simulink model "carboncycle"  (R2020a)
settings: Solver=VariableStepAuto  StartTime=0.0  StopTime=10  RelTol=1e-6
model workspace (MAT data in the model file):
  c_forest_burning_biofuel_co2_released = 1.85
  c_forest_burning_biofuel_energy_released = 4519.72
  c_forest_burning_co2_released = [0.9792 0.9792 2.52 2.52 2.52 2.52 2.52 3.6]
  c_forest_burning_energy_released = [1167.1928 1167.1928 1485.04 1485.04 1485.04 1485.04 1398.78 1398.78]
  c_forest_burning_losses_co2_released = [1.76436 1.76436 0 0 0 0 0 0]
  c_forest_burning_losses_energy_released = [1974.86 1974.86 0 0 0 0 0 0]
  c_harvesting = 1.13940256046
  c_production_biofuel_cost_co2 = 0.74
  c_production_biofuel_cost_tall_oil = 1
  c_production_co2_forest = [0.031 1.667745 0.37375 0.37375 0.37375 0.37375 0.37375 1.1]
  c_production_co2_substitute = [1.539 1.539 1.384806222 1.738255325 12.95940153 13.79703167 0 0]
  c_production_losses_used_for_biofuel = [0 0 0.005521208 0.005521208 0.005521208 0.005521208 0.005521208 0.005521208]
  c_production_losses_used_for_energy = [0.136 0.136 0 0 0 0 0 0]
  c_production_pulp_raw_wood_demand = 3.2229
  c_production_pulp_used = [0 0 1 1 1 1 1 1]
  c_production_pulp_used_reciprocal = [0 0 1 1 1 1 1 1]
  c_production_raw_wood = [2 2 3.2229 3.2229 3.2229 3.2229 3.2229 3.2229]
  c_production_raw_wood_used = [1 1 0 0 0 0 0 0]
  c_production_to_pulp = [0.8 0.8 0 0 0 0 0 0]
  c_recycling_co2_forest = [0 0 1.05 1.05 1.05 1.05 1.05 0]
  c_recycling_co2_substitute = [2.214338235 2.214338235 1.864705882 2.097794118 8.55 0.156 0 0]
  c_substitute_burning_co2_released = [2.922732 2.922732 2.465568 2.773764 0 0 0 0]
  c_substitute_burning_energy_released = [4004.212 4004.212 3616.688 3793.464 0 0 0 0]
  convert_co2_to_forestvolume = 1
  forest_age_0 = 61.5
  forest_area = 20276000
  forest_volume_0 = 2409000000
  initial_stock = 86700000
  k_autotrophic_respiration = 0.5
  k_energy_recovery_forest = [1; 1; 0.070939484; 0.070939484; 0.070939484; 0.070939484; 0.070939484; 1]
  k_energy_recovery_substitute = [0.360473602; 0.360473602; 0.360473602; 0.360473602; 0.111618603; 0; 0; 0]
  k_final_felling = 0.0342
  k_heterotrophic_respiration = 0.5
  k_incineration_forest = [0; 0; 0; 0; 0; 0; 0; 0]
  k_incineration_substitute = [0.008399732; 0.008399732; 0.008399732; 0.008399732; 0.001222426; 0.001; 1; 1]
  k_material_recovery_forest = [0; 0; 0.929060516; 0.929060516; 0.929060516; 0.929060516; 0.929060516; 0]
  k_material_recovery_substitute = [0.631126662; 0.631126662; 0.631126662; 0.631126662; 0.887158971; 0.999; 0; 0]
  k_natural_loss = 0.00227171311509
  k_sustainable_harvesting = 0.03
  k_waste_co2_release_forest = 1
  k_waste_co2_release_substitute = 1
  max_forest = 7227000000
libraries: simulink x3
settings Model: OrderedModelArguments=off  Creator=Cosmo  LastModifiedBy=Roni
settings SolverCC: AlgebraicLoopSolver=LineSearch
settings DataIOCC: SaveFormat=StructureWithTime  SignalLogging=off  DSMLogging=off  SaveTime=off
settings DebuggingCC: ArithmeticOperatorsInVariantConditions=warning
settings SFSimCC: CustomCodeUndefinedFunction=UseInterfaceOnly

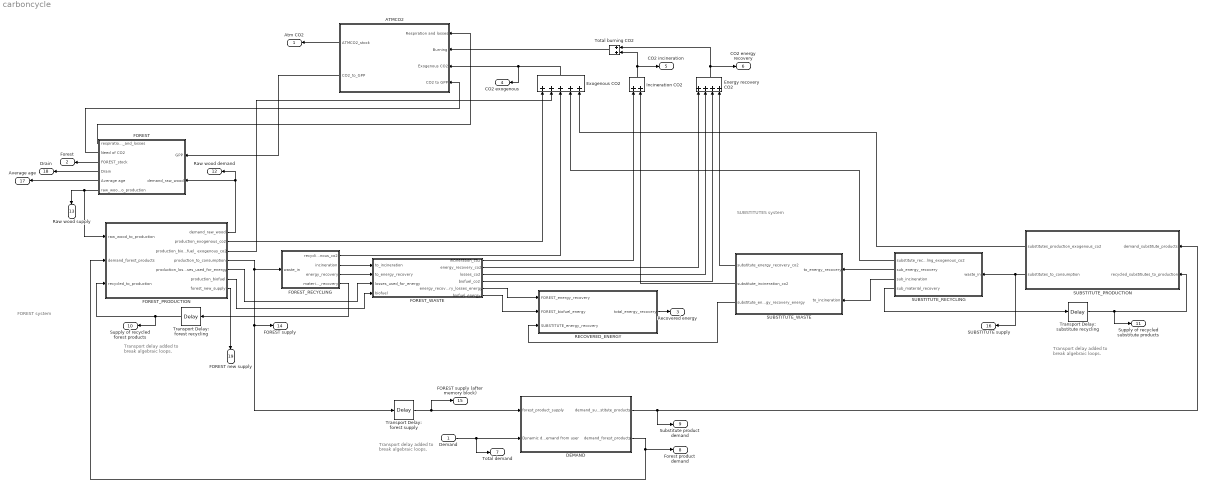
== system carboncycle ==
  note: Transport delay added
      | to break algebraic loops.
  note: FOREST system
  note: SUBSTITUTES system
  note: Transport delay
      | added
      | to break algebraic loops.
  note: Transport delay added
      | to break algebraic loops.
  Demand : Inport  PortDimensions=8
  ATMCO2 : Subsystem
  DEMAND : Subsystem
  Energy recovery CO2 : Sum  Inputs=++++
  Exogenous CO2 : Sum  Inputs=+++++
  FOREST : Subsystem
  FOREST_PRODUCTION : Subsystem
  FOREST_RECYCLING : Subsystem
  FOREST_WASTE : Subsystem
  Incineration CO2 : Sum
  RECOVERED_ENERGY : Subsystem
  SUBSTITUTE_PRODUCTION : Subsystem
  SUBSTITUTE_RECYCLING : Subsystem
  SUBSTITUTE_WASTE : Subsystem
  Total burning CO2 : Sum
  Transport Delay: forest recycling : TransportDelay  DelayTime=0.1
  Transport Delay: forest supply : TransportDelay  DelayTime=0.1
  Transport Delay: substitute recycling : TransportDelay  DelayTime=0.1
  Atm CO2 : Outport
  Forest : Outport  Port=2  Unit=m^3
  Recovered energy : Outport  Port=3
  CO2 exogenous : Outport  Port=4
  CO2 incineration : Outport  Port=5
  CO2 energy recovery : Outport  Port=6
  Total demand : Outport  Port=7
  Forest product demand : Outport  Port=8
  Substitute product demand : Outport  Port=9
  Supply of recycled forest products : Outport  Port=10
  Supply of recycled substitute products : Outport  Port=11
  Raw wood demand : Outport  Port=12
  Raw wood supply : Outport  Port=13
  FOREST supply : Outport  Port=14
  FOREST supply (after memory block) : Outport  Port=15
  SUBSTITUTE supply : Outport  Port=16
  Average age : Outport  Port=17
  Drain : Outport  Port=18  Unit=m^3
  FOREST new supply : Outport  Port=19
  wires:
  ATMCO2/2(CO2_to_GPP) -> FOREST/1(GPP)
  FOREST/1(respiration_and_losses) -> ATMCO2/1(Respiration and losses)
  FOREST/6(raw_wood_to_production) -> Raw wood supply/1, FOREST_PRODUCTION/1(raw_wood_to_production)
  FOREST_RECYCLING/4(material_recovery) -> Transport Delay: forest recycling/1
  FOREST_RECYCLING/1(recycling_exogenous_co2) -> Exogenous CO2/3
  FOREST_PRODUCTION/2(production_exogenous_co2) -> Exogenous CO2/1
  DEMAND/2(demand_forest_products) -> Forest product demand/1, FOREST_PRODUCTION/2(demand_forest_products)
  SUBSTITUTE_PRODUCTION/2(substitutes_to_consumption) -> SUBSTITUTE_RECYCLING/1(waste_in), SUBSTITUTE supply/1
  SUBSTITUTE_RECYCLING/1(substitute_recycling_exogenous_co2) -> Exogenous CO2/4
  SUBSTITUTE_PRODUCTION/1(substitutes_production_exogenous_co2) -> Exogenous CO2/5
  SUBSTITUTE_WASTE/1(substitute_energy_recovery_co2) -> Energy recovery CO2/4
  SUBSTITUTE_RECYCLING/4(sub_material_recovery) -> Transport Delay: substitute recycling/1
  FOREST/2(Need of CO2) -> ATMCO2/4(CO2 to GPP)
  FOREST_RECYCLING/2(incineration) -> FOREST_WASTE/1(to_incineration)
  FOREST_RECYCLING/3(energy_recovery) -> FOREST_WASTE/2(to_energy_recovery)
  FOREST_WASTE/1(incineration_co2) -> Incineration CO2/1
  FOREST_WASTE/5(energy_recovery_losses_energy) -> RECOVERED_ENERGY/1(FOREST_energy_recovery)
  RECOVERED_ENERGY/1(total_energy_recovery) -> Recovered energy/1
  SUBSTITUTE_WASTE/3(substitute_energy_recovery_energy) -> RECOVERED_ENERGY/3(SUBSTITUTE_energy_recovery)
  FOREST_WASTE/2(energy_recovery_co2) -> Energy recovery CO2/1
  Incineration CO2/1 -> CO2 incineration/1, Total burning CO2/2
  Total burning CO2/1 -> ATMCO2/2(Burning)
  SUBSTITUTE_RECYCLING/2(sub_energy_recovery) -> SUBSTITUTE_WASTE/1(to_energy_recovery)
  SUBSTITUTE_RECYCLING/3(sub_incineration) -> SUBSTITUTE_WASTE/2(to_incineration)
  Transport Delay: forest recycling/1 -> Supply of recycled forest products/1, FOREST_PRODUCTION/3(recycled_to_production)
  Energy recovery CO2/1 -> CO2 energy recovery/1, Total burning CO2/1
  Exogenous CO2/1 -> CO2 exogenous/1, ATMCO2/3(Exogenous CO2)
  Transport Delay: forest supply/1 -> FOREST supply (after memory block)/1, DEMAND/1(forest_product_supply)
  FOREST_PRODUCTION/4(production_to_consumption) -> Transport Delay: forest supply/1, FOREST supply/1, FOREST_RECYCLING/1(waste_in)
  Transport Delay: substitute recycling/1 -> Supply of recycled substitute products/1, SUBSTITUTE_PRODUCTION/2(recycled_substitiutes_to_production)
  FOREST/3(FOREST_stock) -> Forest/1
  ATMCO2/1(ATMCO2_stock) -> Atm CO2/1
  FOREST_PRODUCTION/1(demand_raw_wood) -> Raw wood demand/1, FOREST/2(demand_raw_wood)
  FOREST_PRODUCTION/5(production_losses_used_for_energy) -> FOREST_WASTE/3(losses_used_for_energy)
  FOREST_PRODUCTION/6(production_biofuel) -> FOREST_WASTE/4(biofuel)
  FOREST_PRODUCTION/3(production_biofuel_ exogenous_co2) -> Exogenous CO2/2
  FOREST_WASTE/6(biofuel_energy) -> RECOVERED_ENERGY/2(FOREST_biofuel_energy)
  FOREST_WASTE/3(losses_co2) -> Energy recovery CO2/2
  FOREST_WASTE/4(biofuel_co2) -> Energy recovery CO2/3
  SUBSTITUTE_WASTE/2(substitute_incineration_co2) -> Incineration CO2/2
  FOREST/5(Average age) -> Average age/1
  FOREST/4(Drain) -> Drain/1
  DEMAND/1(demand_substitute_products) -> Substitute product demand/1, SUBSTITUTE_PRODUCTION/1(demand_substitute_products)
  Demand/1 -> Total demand/1, DEMAND/2(Dynamic demand from user)
  FOREST_PRODUCTION/7(forest_new_supply) -> FOREST new supply/1

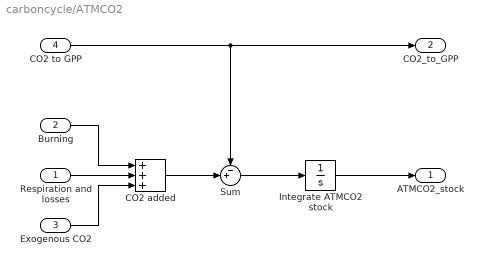
== system carboncycle/ATMCO2 ==
  Respiration and losses : Inport
  Burning : Inport  Port=2
  Exogenous CO2 : Inport  Port=3  Unit=t
  CO2 to GPP : Inport  Port=4  Unit=t
  CO2 added : Sum  Inputs=+++
  Integrate ATMCO2 stock : Integrator
  Sum : Sum  Inputs=-+|
  ATMCO2_stock : Outport  Unit=t
  CO2_to_GPP : Outport  Port=2  Unit=t
  wires:
  Burning/1 -> CO2 added/1
  Respiration and losses/1 -> CO2 added/2
  Exogenous CO2/1 -> CO2 added/3
  Integrate ATMCO2 stock/1 -> ATMCO2_stock/1
  Sum/1 -> Integrate ATMCO2 stock/1
  CO2 added/1 -> Sum/2
  CO2 to GPP/1 -> Sum/1, CO2_to_GPP/1

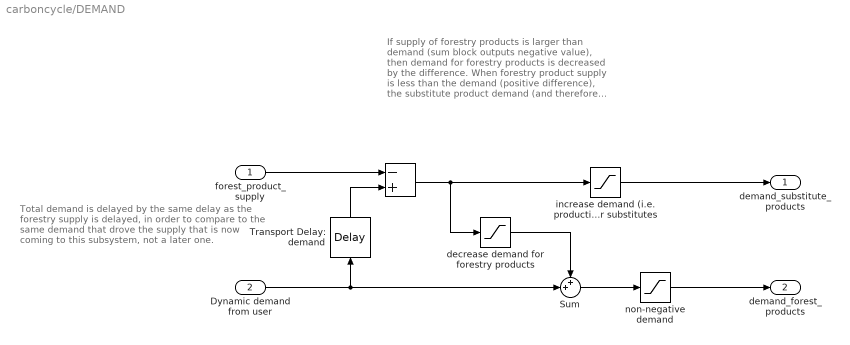
== system carboncycle/DEMAND ==
  note: If supply of forestry products is larger than demand (sum block outputs negative value), then demand for forestry products is decreased by the difference.
      |
      | When forestry product supply is less than the demand (positive difference), the substitute product demand (and therefore production) is equal to this difference.
  note: Total demand is delayed by the same delay as the forestry supply is delayed, in order to compare to the same demand that drove the supply that is now coming to this subsystem, not a later one.
  forest_product_supply : Inport
  Dynamic demand from user : Inport  Port=2
  " " : Sum  Inputs=-+
  Sum : Sum  Inputs=++|
  Transport Delay: demand : TransportDelay  DelayTime=0.1
  decrease demand for forestry products : Saturate  UpperLimit=0  LowerLimit=-inf  ZeroCross=off
  increase demand (i.e. production) for substitutes : Saturate  UpperLimit=inf  LowerLimit=0  ZeroCross=off
  non-negative demand : Saturate  UpperLimit=inf  LowerLimit=0
  demand_substitute_products : Outport
  demand_forest_products : Outport  Port=2
  wires:
  " "/1 -> decrease demand for forestry products/1, increase demand (i.e. production) for substitutes/1
  decrease demand for forestry products/1 -> Sum/1
  Sum/1 -> non-negative demand/1
  forest_product_supply/1 -> " "/1
  Dynamic demand from user/1 -> Sum/2, Transport Delay: demand/1
  non-negative demand/1 -> demand_forest_products/1
  increase demand (i.e. production) for substitutes/1 -> demand_substitute_products/1
  Transport Delay: demand/1 -> " "/2

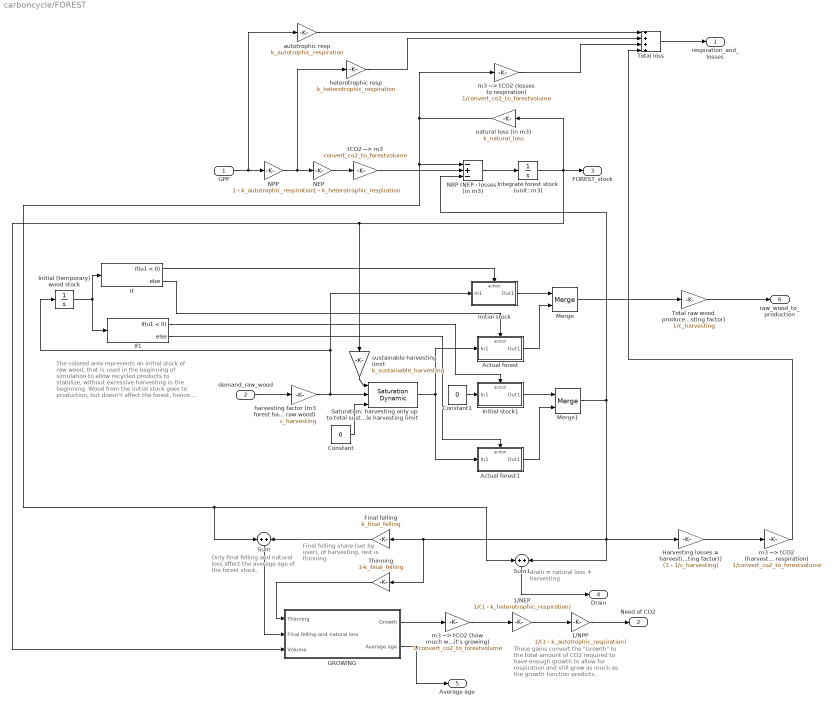
== system carboncycle/FOREST ==
  note: drain =
      | natural loss
      | + harvesting
  note: Final felling share (set
      | by user), of harvesting,
      | rest is thinning.
  note: The colored area represents an initial stock of raw wood, that is used in the beginning of simulation to allow recycled products to stabilize, without excessive harvesting in the beginning. Wood from the initial stock goes to production, but doesn't affect the forest, hence different merge blocks.
      |
      | After the initial stock is empty (i.e. u1 > 0), we start to harvest the actual forest.
  note: Only final felling
      | and natural loss
      | affect the average
      | age of the forest
      | stock.
  note: These gains convert the "Growth"
      | to the total amount of CO2 required
      | to have enough growth to allow for
      | respiration and still grow as much as
      | the growth function predicts.
  GPP : Inport
  demand_raw_wood : Inport  Port=2  Unit=m^3
  1/NEP : Gain  Gain=1/(1 - k_heterotrophic_respiration)
  1/NPP : Gain  Gain=1/(1 - k_autotrophic_respiration)
  Actual forest : Subsystem  TreatAsAtomicUnit=on
  Actual forest1 : Subsystem  TreatAsAtomicUnit=on
  Constant : Constant  Value=0
  Constant1 : Constant  Value=0
  Final felling : Gain  Gain=k_final_felling
  GROWING : Subsystem
  Harvesting losses = harvesting * (1 - 1 / (harvesting factor)) : Gain  Gain=(1 - 1/c_harvesting)
  If : If  IfExpression=u1 < 0  ZeroCross=off
  If1 : If  IfExpression=u1 < 0  ZeroCross=off
  Initial (temporary) wood stock : Integrator  InitialCondition=-initial_stock
  Initial stock : Subsystem  TreatAsAtomicUnit=on
  Initial stock1 : Subsystem  TreatAsAtomicUnit=on
  Integrate forest stock (unit: m3) : Integrator  InitialCondition=forest_volume_0
  Merge : Merge
  Merge1 : Merge
  NBP (NEP - losses) (in m3) : Sum  Inputs=-+-
  NEP : Gain  Gain=1 - k_heterotrophic_respiration
  NPP : Gain  Gain=1 - k_autotrophic_respiration
  Saturation: harvesting only up to total sustainable harvesting limit : simulink/Discontinuities/Saturation Dynamic  OutMin=[]  OutMax=[]  OutDataTypeStr=Inherit: Same as second input  OutDataType=fixdt(1, 16)  OutScaling=2^-10  DoSatur=off
  Sum : Sum  Inputs=+|+
  Sum1 : Sum  Inputs=+|+
  Thinning : Gain  Gain=1-k_final_felling
  Total loss : Sum  Inputs=++++
  Total raw wood produced = harvesting / (harvesting factor) : Gain  Gain=1/c_harvesting
  autotrophic resp : Gain  Gain=k_autotrophic_respiration
  harvesting factor (m3 forest harvested for m3 raw wood) : Gain  Gain=c_harvesting
  heterotrophic resp : Gain  Gain=k_heterotrophic_respiration
  m3 --> tCO2 (harvesting losses to respiration) : Gain  Gain=1/convert_co2_to_forestvolume
  m3 --> tCO2 (how much wood absorbs CO2 when it's growing) : Gain  Gain=1/convert_co2_to_forestvolume
  m3 --> tCO2 (losses to respiration) : Gain  Gain=1/convert_co2_to_forestvolume
  natural loss (in m3) : Gain  Gain=k_natural_loss
  sustainable harvesting limit : Gain  Gain=k_sustainable_harvesting
  tCO2 --> m3 : Gain  Gain=convert_co2_to_forestvolume
  respiration_and_losses : Outport  Unit=t
  Need of CO2 : Outport  Port=2  Unit=t  VectorParamsAs1DForOutWhenUnconnected=off
  FOREST_stock : Outport  Port=3  Unit=m^3
  Drain : Outport  Port=4  Unit=m^3
  Average age : Outport  Port=5  Unit=y  VectorParamsAs1DForOutWhenUnconnected=off
  raw_wood_to_production : Outport  Port=6  Unit=m^3
  wires:
  GPP/1 -> autotrophic resp/1, NPP/1
  NPP/1 -> heterotrophic resp/1, NEP/1
  NEP/1 -> tCO2 --> m3/1
  autotrophic resp/1 -> Total loss/1
  heterotrophic resp/1 -> Total loss/2
  Total loss/1 -> respiration_and_losses/1
  NBP (NEP - losses) (in m3)/1 -> Integrate forest stock (unit: m3)/1
  natural loss (in m3)/1 -> Sum1/1, Sum/1, NBP (NEP - losses) (in m3)/1, m3 --> tCO2 (losses to respiration)/1
  demand_raw_wood/1 -> harvesting factor (m3 forest harvested for m3 raw wood)/1
  Total raw wood produced = harvesting / (harvesting factor)/1 -> raw_wood_to_production/1
  tCO2 --> m3/1 -> NBP (NEP - losses) (in m3)/2
  m3 --> tCO2 (losses to respiration)/1 -> Total loss/3
  Harvesting losses = harvesting * (1 - 1 / (harvesting factor))/1 -> m3 --> tCO2 (harvesting losses to respiration)/1
  m3 --> tCO2 (harvesting losses to respiration)/1 -> Total loss/4
  m3 --> tCO2 (how much wood absorbs CO2 when it's growing)/1 -> 1/NEP/1
  1/NPP/1 -> Need of CO2/1
  1/NEP/1 -> 1/NPP/1
  GROWING/1("Growth ") -> m3 --> tCO2 (how much wood absorbs CO2 when it's growing)/1
  Integrate forest stock (unit: m3)/1 -> natural loss (in m3)/1, FOREST_stock/1, sustainable harvesting limit/1, GROWING/3(Volume)
  Thinning/1 -> GROWING/1(Thinning)
  Sum/1 -> GROWING/2("Final felling and natural loss ")
  Final felling/1 -> Sum/2
  GROWING/2(Average age) -> Average age/1
  Constant/1 -> Saturation: harvesting only up to total sustainable harvesting limit/3
  harvesting factor (m3 forest harvested for m3 raw wood)/1 -> Initial (temporary) wood stock/1, Initial stock/1(In1), Saturation: harvesting only up to total sustainable harvesting limit/2
  Initial (temporary) wood stock/1 -> If/1, If1/1
  sustainable harvesting limit/1 -> Saturation: harvesting only up to total sustainable harvesting limit/1
  If/1 -> Initial stock/Action
  If/2 -> Actual forest/Action
  Saturation: harvesting only up to total sustainable harvesting limit/1 -> Actual forest/1(In1), Actual forest1/1(In1)
  Initial stock/1(Out1) -> Merge/1
  Merge/1 -> Total raw wood produced = harvesting / (harvesting factor)/1
  Actual forest/1(Out1) -> Merge/2
  Merge1/1 -> NBP (NEP - losses) (in m3)/3, Thinning/1, Final felling/1, Sum1/2, Harvesting losses = harvesting * (1 - 1 / (harvesting factor))/1
  Actual forest1/1(Out1) -> Merge1/2
  Initial stock1/1(Out1) -> Merge1/1
  If1/1 -> Initial stock1/Action
  Constant1/1 -> Initial stock1/1(In1)
  If1/2 -> Actual forest1/Action
  Sum1/1 -> Drain/1

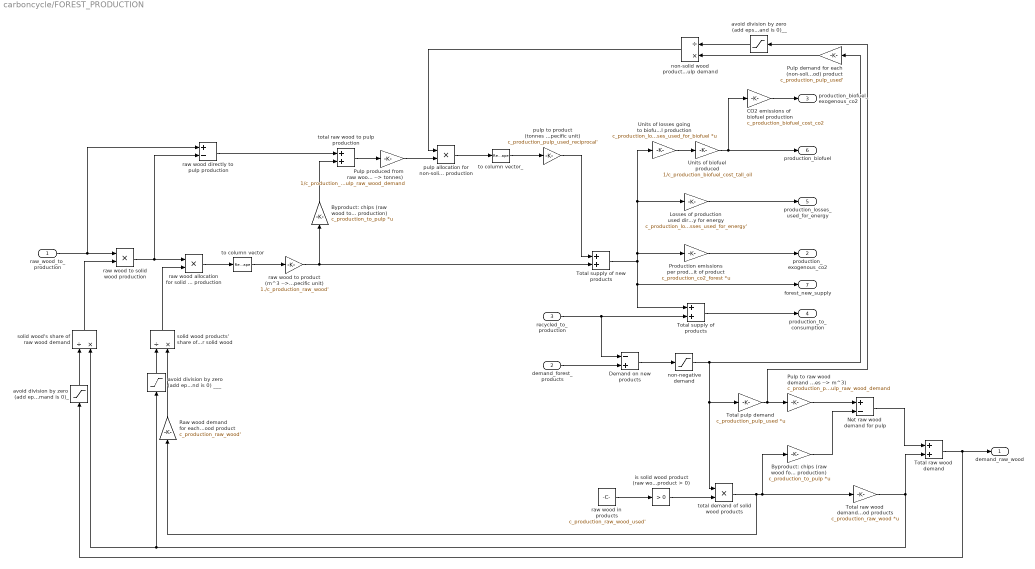
== system carboncycle/FOREST_PRODUCTION ==
  raw_wood_to_production : Inport  Unit=m^3
  demand_forest_products : Inport  Port=2
  recycled_to_production : Inport  Port=3
  Byproduct: chips (raw wood for pulp production) : Gain  Gain=c_production_to_pulp  Multiplication=Matrix(K*u)
  Byproduct: chips (raw wood to pulp production) : Gain  Gain=c_production_to_pulp  Multiplication=Matrix(K*u)
  CO2 emissions of biofuel production : Gain  Gain=c_production_biofuel_cost_co2
  Demand on new products : Sum  Inputs=-+
  Losses of production used directly for energy : Gain  Gain=c_production_losses_used_for_energy'
  Net raw wood demand for pulp : Sum  Inputs=+-
  Production emissions per produced unit of product : Gain  Gain=c_production_co2_forest  Multiplication=Matrix(K*u)
  Pulp demand for each (non-solid wood) product : Gain  Gain=c_production_pulp_used'
  Pulp produced from raw wood (m^3 --> tonnes) : Gain  Gain=1/c_production_pulp_raw_wood_demand
  Pulp to raw wood demand (tonnes --> m^3) : Gain  Gain=c_production_pulp_raw_wood_demand
  Raw wood demand for each solid wood product : Gain  Gain=c_production_raw_wood'
  Total pulp demand : Gain  Gain=c_production_pulp_used  Multiplication=Matrix(K*u)
  Total raw wood demand : Sum
  Total raw wood demand for solid wood products : Gain  Gain=c_production_raw_wood  Multiplication=Matrix(K*u)
  Total supply of new products : Sum
  Total supply of products : Sum
  Units of biofuel produced : Gain  Gain=1/c_production_biofuel_cost_tall_oil
  Units of losses going to biofuel production : Gain  Gain=c_production_losses_used_for_biofuel  Multiplication=Matrix(K*u)
  avoid division by zero (add eps if total demand is 0)_ : Saturate  UpperLimit=Inf  LowerLimit=eps
  avoid division by zero (add eps if total demand is 0)__ : Saturate  UpperLimit=Inf  LowerLimit=eps
  avoid division by zero (add eps if total demand is 0) ___ : Saturate  UpperLimit=Inf  LowerLimit=eps
  is solid wood product (raw wood in product > 0) : simulink/Logic and Bit Operations/Compare To Zero  relop=>  OutDataTypeStr=boolean
  non-negative demand : Saturate  UpperLimit=Inf  LowerLimit=0
  non-solid wood products' share of pulp demand : Product  Inputs=/*  OutMin=0  OutMax=1
  pulp allocation for non-solid wood production : Product
  pulp to product (tonnes --> product- specific unit) : Gain  Gain=c_production_pulp_used_reciprocal'
  raw wood allocation for solid wood production : Product
  raw wood directly to pulp production : Sum  Inputs=+-
  raw wood in products : Constant  Value=c_production_raw_wood_used'
  raw wood to product (m^3 --> product-specific unit) : Gain  Gain=1./c_production_raw_wood'
  raw wood to solid wood production : Product
  solid wood products' share of raw wood demand for solid wood : Product  Inputs=/*  OutMin=0  OutMax=1
  solid wood's share of raw wood demand : Product  Inputs=/*  OutMin=0  OutMax=1
  to column vector : Reshape  OutputDimensionality=Column vector (2-D)
  to column vector_ : Reshape  OutputDimensionality=Column vector (2-D)
  total demand of solid wood products : Product  OutDataTypeStr=double
  total raw wood to pulp production : Sum
  demand_raw_wood : Outport  Unit=m^3
  production_exogenous_co2 : Outport  Port=2  Unit=t
  production_biofuel_ exogenous_co2 : Outport  Port=3  Unit=t
  production_to_consumption : Outport  Port=4
  production_losses_used_for_energy : Outport  Port=5
  production_biofuel : Outport  Port=6
  forest_new_supply : Outport  Port=7
  wires:
  Production emissions per produced unit of product/1 -> production_exogenous_co2/1
  Total supply of products/1 -> production_to_consumption/1
  raw_wood_to_production/1 -> raw wood to solid wood production/1, raw wood directly to pulp production/1
  Demand on new products/1 -> non-negative demand/1
  demand_forest_products/1 -> Demand on new products/2
  recycled_to_production/1 -> Demand on new products/1, Total supply of products/2
  non-negative demand/1 -> total demand of solid wood products/1, Total pulp demand/1, Pulp demand for each (non-solid wood) product/1
  is solid wood product (raw wood in product > 0)/1 -> total demand of solid wood products/2
  raw wood in products/1 -> is solid wood product (raw wood in product > 0)/1
  total demand of solid wood products/1 -> Byproduct: chips (raw wood for pulp production)/1, Total raw wood demand for solid wood products/1, Raw wood demand for each solid wood product/1
  Total pulp demand/1 -> avoid division by zero (add eps if total demand is 0)__/1, Pulp to raw wood demand (tonnes --> m^3)/1
  Pulp to raw wood demand (tonnes --> m^3)/1 -> Net raw wood demand for pulp/1
  Byproduct: chips (raw wood for pulp production)/1 -> Net raw wood demand for pulp/2
  Net raw wood demand for pulp/1 -> Total raw wood demand/1
  Total raw wood demand for solid wood products/1 -> Total raw wood demand/2, solid wood's share of raw wood demand/2, avoid division by zero (add eps if total demand is 0) ___/1
  Total raw wood demand/1 -> avoid division by zero (add eps if total demand is 0)_/1, demand_raw_wood/1
  avoid division by zero (add eps if total demand is 0)_/1 -> solid wood's share of raw wood demand/1
  solid wood's share of raw wood demand/1 -> raw wood to solid wood production/2
  raw wood to solid wood production/1 -> raw wood allocation for solid wood production/1, raw wood directly to pulp production/2
  raw wood to product (m^3 --> product-specific unit)/1 -> Total supply of new products/2, Byproduct: chips (raw wood to pulp production)/1
  Byproduct: chips (raw wood to pulp production)/1 -> total raw wood to pulp production/2
  raw wood directly to pulp production/1 -> total raw wood to pulp production/1
  Raw wood demand for each solid wood product/1 -> solid wood products' share of raw wood demand for solid wood/2
  avoid division by zero (add eps if total demand is 0) ___/1 -> solid wood products' share of raw wood demand for solid wood/1
  solid wood products' share of raw wood demand for solid wood/1 -> raw wood allocation for solid wood production/2
  raw wood allocation for solid wood production/1 -> to column vector/1
  total raw wood to pulp production/1 -> Pulp produced from raw wood (m^3 --> tonnes)/1
  pulp to product (tonnes --> product- specific unit)/1 -> Total supply of new products/1
  to column vector/1 -> raw wood to product (m^3 --> product-specific unit)/1
  Pulp produced from raw wood (m^3 --> tonnes)/1 -> pulp allocation for non-solid wood production/2
  pulp allocation for non-solid wood production/1 -> to column vector_/1
  to column vector_/1 -> pulp to product (tonnes --> product- specific unit)/1
  avoid division by zero (add eps if total demand is 0)__/1 -> non-solid wood products' share of pulp demand/1
  Pulp demand for each (non-solid wood) product/1 -> non-solid wood products' share of pulp demand/2
  non-solid wood products' share of pulp demand/1 -> pulp allocation for non-solid wood production/1
  Losses of production used directly for energy/1 -> production_losses_used_for_energy/1
  Units of losses going to biofuel production/1 -> Units of biofuel produced/1
  Total supply of new products/1 -> Units of losses going to biofuel production/1, Losses of production used directly for energy/1, Production emissions per produced unit of product/1, Total supply of products/1, forest_new_supply/1
  Units of biofuel produced/1 -> CO2 emissions of biofuel production/1, production_biofuel/1
  CO2 emissions of biofuel production/1 -> production_biofuel_ exogenous_co2/1

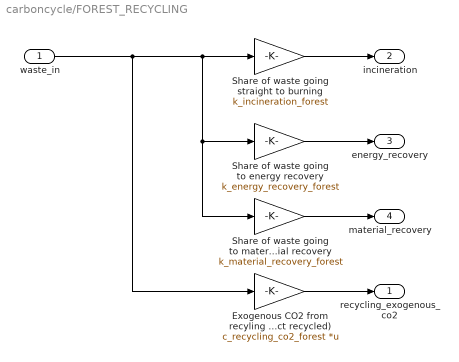
== system carboncycle/FOREST_RECYCLING ==
  waste_in : Inport
  Exogenous CO2 from recyling (tCO2 / unit of product recycled) : Gain  Gain=c_recycling_co2_forest  Multiplication=Matrix(K*u)
  Share of waste going straight to burning : Gain  Gain=k_incineration_forest
  Share of waste going to energy recovery : Gain  Gain=k_energy_recovery_forest
  Share of waste going to material recovery : Gain  Gain=k_material_recovery_forest
  recycling_exogenous_co2 : Outport  Unit=t
  incineration : Outport  Port=2
  energy_recovery : Outport  Port=3
  material_recovery : Outport  Port=4
  wires:
  Share of waste going to material recovery/1 -> material_recovery/1
  Exogenous CO2 from recyling (tCO2 / unit of product recycled)/1 -> recycling_exogenous_co2/1
  Share of waste going to energy recovery/1 -> energy_recovery/1
  waste_in/1 -> Exogenous CO2 from recyling (tCO2 / unit of product recycled)/1, Share of waste going to energy recovery/1, Share of waste going to material recovery/1, Share of waste going straight to burning/1
  Share of waste going straight to burning/1 -> incineration/1

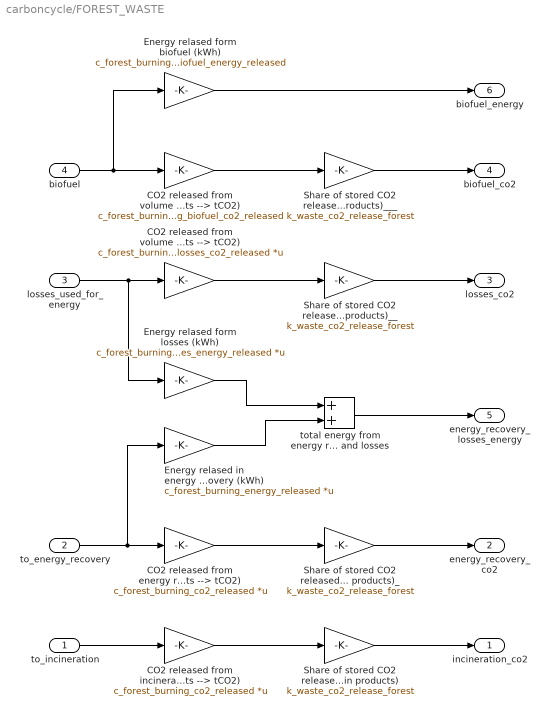
== system carboncycle/FOREST_WASTE ==
  to_incineration : Inport
  to_energy_recovery : Inport  Port=2
  losses_used_for_energy : Inport  Port=3
  biofuel : Inport  Port=4
  CO2 released from energy recovery volume (product units --> tCO2) : Gain  Gain=c_forest_burning_co2_released  Multiplication=Matrix(K*u)
  CO2 released from incineration volume (product units --> tCO2) : Gain  Gain=c_forest_burning_co2_released  Multiplication=Matrix(K*u)
  CO2 released from volume of biofuel (biofuel units --> tCO2) : Gain  Gain=c_forest_burning_biofuel_co2_released
  CO2 released from volume of losses used for energy (loss units --> tCO2) : Gain  Gain=c_forest_burning_losses_co2_released  Multiplication=Matrix(K*u)
  Energy relased form biofuel (kWh) : Gain  Gain=c_forest_burning_biofuel_energy_released
  Energy relased form losses (kWh) : Gain  Gain=c_forest_burning_losses_energy_released  Multiplication=Matrix(K*u)
  Energy relased in energy recovery (kWh) : Gain  Gain=c_forest_burning_energy_released  Multiplication=Matrix(K*u)
  Share of stored CO2 released through burning (tCO2 / tCO2 stored in products) : Gain  Gain=k_waste_co2_release_forest
  Share of stored CO2 released through burning (tCO2 / tCO2 stored in products)_ : Gain  Gain=k_waste_co2_release_forest
  Share of stored CO2 released through burning (tCO2 / tCO2 stored in products)__ : Gain  Gain=k_waste_co2_release_forest
  Share of stored CO2 released through burning (tCO2 / tCO2 stored in products)___ : Gain  Gain=k_waste_co2_release_forest
  total energy from energy recovery and losses : Sum
  incineration_co2 : Outport  Unit=t
  energy_recovery_co2 : Outport  Port=2  Unit=t
  losses_co2 : Outport  Port=3  Unit=t
  biofuel_co2 : Outport  Port=4  Unit=t
  energy_recovery_losses_energy : Outport  Port=5  Unit=kWh
  biofuel_energy : Outport  Port=6  Unit=kWh
  wires:
  CO2 released from incineration volume (product units --> tCO2)/1 -> Share of stored CO2 released through burning (tCO2 / tCO2 stored in products)/1
  Share of stored CO2 released through burning (tCO2 / tCO2 stored in products)/1 -> incineration_co2/1
  to_energy_recovery/1 -> CO2 released from energy recovery volume (product units --> tCO2)/1, Energy relased in energy recovery (kWh)/1
  to_incineration/1 -> CO2 released from incineration volume (product units --> tCO2)/1
  CO2 released from energy recovery volume (product units --> tCO2)/1 -> Share of stored CO2 released through burning (tCO2 / tCO2 stored in products)_/1
  Share of stored CO2 released through burning (tCO2 / tCO2 stored in products)_/1 -> energy_recovery_co2/1
  losses_used_for_energy/1 -> Energy relased form losses (kWh)/1, CO2 released from volume of losses used for energy (loss units --> tCO2)/1
  CO2 released from volume of losses used for energy (loss units --> tCO2)/1 -> Share of stored CO2 released through burning (tCO2 / tCO2 stored in products)__/1
  CO2 released from volume of biofuel (biofuel units --> tCO2)/1 -> Share of stored CO2 released through burning (tCO2 / tCO2 stored in products)___/1
  biofuel/1 -> Energy relased form biofuel (kWh)/1, CO2 released from volume of biofuel (biofuel units --> tCO2)/1
  Share of stored CO2 released through burning (tCO2 / tCO2 stored in products)___/1 -> biofuel_co2/1
  Share of stored CO2 released through burning (tCO2 / tCO2 stored in products)__/1 -> losses_co2/1
  Energy relased in energy recovery (kWh)/1 -> total energy from energy recovery and losses/2
  Energy relased form losses (kWh)/1 -> total energy from energy recovery and losses/1
  total energy from energy recovery and losses/1 -> energy_recovery_losses_energy/1
  Energy relased form biofuel (kWh)/1 -> biofuel_energy/1

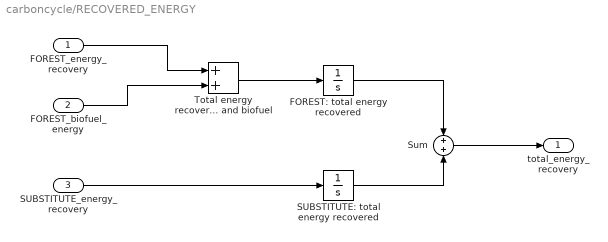
== system carboncycle/RECOVERED_ENERGY ==
  FOREST_energy_recovery : Inport  Unit=kWh
  FOREST_biofuel_energy : Inport  Port=2  Unit=kWh
  SUBSTITUTE_energy_recovery : Inport  Port=3  Unit=kWh
  FOREST: total energy recovered : Integrator
  SUBSTITUTE: total energy recovered : Integrator
  Sum : Sum
  "Total energy recovered from forest products, production (losses) and biofuel" : Sum
  total_energy_recovery : Outport
  wires:
  FOREST: total energy recovered/1 -> Sum/1
  SUBSTITUTE_energy_recovery/1 -> SUBSTITUTE: total energy recovered/1
  SUBSTITUTE: total energy recovered/1 -> Sum/2
  Sum/1 -> total_energy_recovery/1
  FOREST_energy_recovery/1 -> "Total energy recovered from forest products, production (losses) and biofuel"/1
  "Total energy recovered from forest products, production (losses) and biofuel"/1 -> FOREST: total energy recovered/1
  FOREST_biofuel_energy/1 -> "Total energy recovered from forest products, production (losses) and biofuel"/2

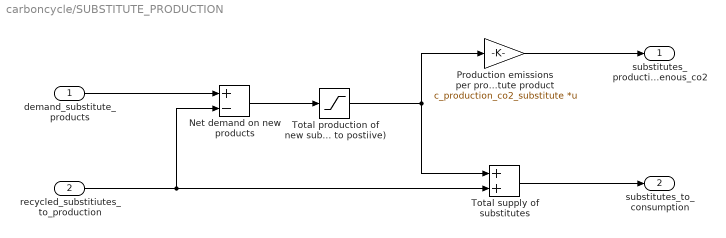
== system carboncycle/SUBSTITUTE_PRODUCTION ==
  demand_substitute_products : Inport
  recycled_substitiutes_to_production : Inport  Port=2
  Net demand on new products : Sum  Inputs=+-
  Production emissions per produced unit of substitute product : Gain  Gain=c_production_co2_substitute  Multiplication=Matrix(K*u)
  Total production of new substitute products (saturate to postiive) : Saturate  UpperLimit=inf  LowerLimit=0  ZeroCross=off
  Total supply of substitutes : Sum
  substitutes_production_exogenous_co2 : Outport  Unit=t
  substitutes_to_consumption : Outport  Port=2
  wires:
  Production emissions per produced unit of substitute product/1 -> substitutes_production_exogenous_co2/1
  Net demand on new products/1 -> Total production of new substitute products (saturate to postiive)/1
  demand_substitute_products/1 -> Net demand on new products/1
  recycled_substitiutes_to_production/1 -> Net demand on new products/2, Total supply of substitutes/2
  Total production of new substitute products (saturate to postiive)/1 -> Total supply of substitutes/1, Production emissions per produced unit of substitute product/1
  Total supply of substitutes/1 -> substitutes_to_consumption/1

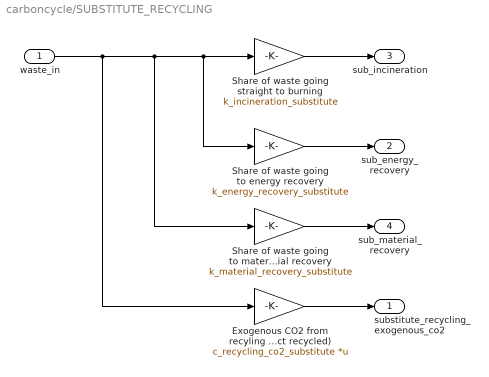
== system carboncycle/SUBSTITUTE_RECYCLING ==
  waste_in : Inport
  Exogenous CO2 from recyling (tCO2 / unit of product recycled) : Gain  Gain=c_recycling_co2_substitute  Multiplication=Matrix(K*u)
  Share of waste going straight to burning : Gain  Gain=k_incineration_substitute
  Share of waste going to energy recovery : Gain  Gain=k_energy_recovery_substitute
  Share of waste going to material recovery : Gain  Gain=k_material_recovery_substitute
  substitute_recycling_exogenous_co2 : Outport  Unit=t
  sub_energy_recovery : Outport  Port=2
  sub_incineration : Outport  Port=3
  sub_material_recovery : Outport  Port=4
  wires:
  Exogenous CO2 from recyling (tCO2 / unit of product recycled)/1 -> substitute_recycling_exogenous_co2/1
  Share of waste going to material recovery/1 -> sub_material_recovery/1
  waste_in/1 -> Exogenous CO2 from recyling (tCO2 / unit of product recycled)/1, Share of waste going to energy recovery/1, Share of waste going straight to burning/1, Share of waste going to material recovery/1
  Share of waste going straight to burning/1 -> sub_incineration/1
  Share of waste going to energy recovery/1 -> sub_energy_recovery/1

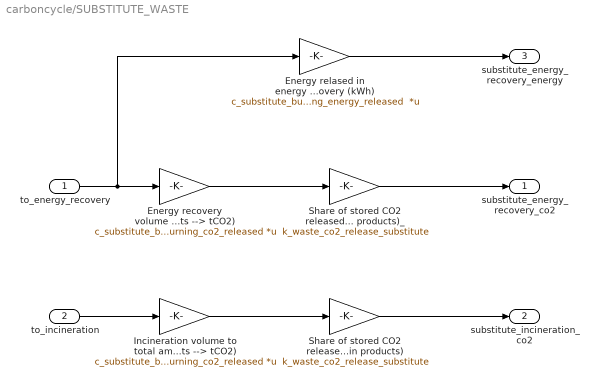
== system carboncycle/SUBSTITUTE_WASTE ==
  to_energy_recovery : Inport
  to_incineration : Inport  Port=2
  Energy recovery volume to total amount of CO2 relesead from products (product units --> tCO2) : Gain  Gain=c_substitute_burning_co2_released  Multiplication=Matrix(K*u)
  Energy relased in energy recovery (kWh) : Gain  Gain=c_substitute_burning_energy_released  Multiplication=Matrix(K*u)
  Incineration volume to total amount of CO2 released from products (product units --> tCO2) : Gain  Gain=c_substitute_burning_co2_released  Multiplication=Matrix(K*u)
  Share of stored CO2 released through burning (tCO2 / tCO2 stored in products) : Gain  Gain=k_waste_co2_release_substitute
  Share of stored CO2 released through burning (tCO2 / tCO2 stored in products)_ : Gain  Gain=k_waste_co2_release_substitute
  substitute_energy_recovery_co2 : Outport  Unit=t
  substitute_incineration_co2 : Outport  Port=2  Unit=t
  substitute_energy_recovery_energy : Outport  Port=3  Unit=kWh
  wires:
  Share of stored CO2 released through burning (tCO2 / tCO2 stored in products)_/1 -> substitute_energy_recovery_co2/1
  to_energy_recovery/1 -> Energy relased in energy recovery (kWh)/1, Energy recovery volume to total amount of CO2 relesead from products (product units --> tCO2)/1
  Energy recovery volume to total amount of CO2 relesead from products (product units --> tCO2)/1 -> Share of stored CO2 released through burning (tCO2 / tCO2 stored in products)_/1
  Incineration volume to total amount of CO2 released from products (product units --> tCO2)/1 -> Share of stored CO2 released through burning (tCO2 / tCO2 stored in products)/1
  to_incineration/1 -> Incineration volume to total amount of CO2 released from products (product units --> tCO2)/1
  Share of stored CO2 released through burning (tCO2 / tCO2 stored in products)/1 -> substitute_incineration_co2/1
  Energy relased in energy recovery (kWh)/1 -> substitute_energy_recovery_energy/1

== system carboncycle/FOREST/Actual forest ==
  In1 : Inport
  Action Port : ActionPort  ActionPortLabel=else
  Out1 : Outport
  wires:
  In1/1 -> Out1/1

== system carboncycle/FOREST/Actual forest1 ==
  In1 : Inport
  Action Port : ActionPort  ActionPortLabel=else
  Out1 : Outport
  wires:
  In1/1 -> Out1/1

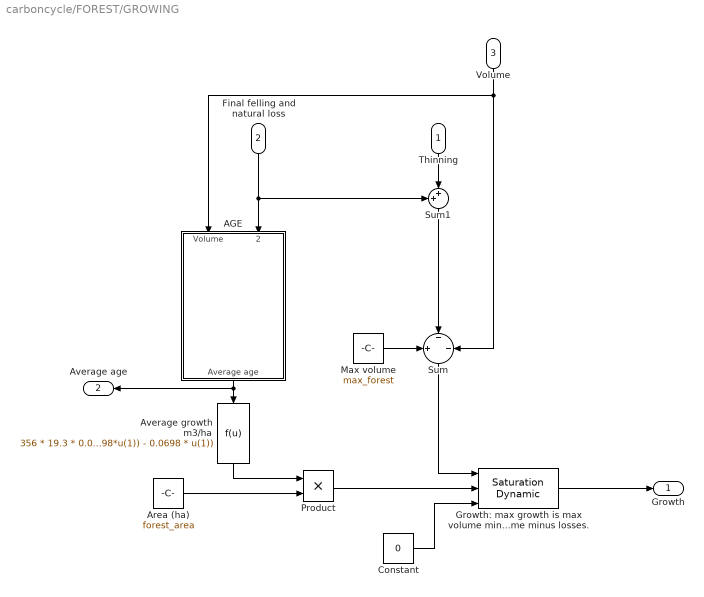
== system carboncycle/FOREST/GROWING ==
  Thinning : Inport
  "Final felling and natural loss " : Inport  Port=2
  Volume : Inport  Port=3
  AGE : Subsystem
  Area (ha) : Constant  Value=forest_area
  Average growth m3/ha : Fcn  Expr=356 * 19.3 * 0.0698 * exp(-19.3 * exp(-0.0698*u(1)) - 0.0698 * u(1))
  Constant : Constant  Value=0
  Growth: max growth is max volume minus current volume minus losses. : simulink/Discontinuities/Saturation Dynamic  OutMin=[]  OutMax=[]  OutDataTypeStr=Inherit: Same as second input  OutDataType=fixdt(1, 16)  OutScaling=2^-10  DoSatur=off
  Max volume : Constant  Value=max_forest
  Product : Product
  Sum : Sum  Inputs=+|-|-
  Sum1 : Sum  Inputs=++|
  "Growth " : Outport  VectorParamsAs1DForOutWhenUnconnected=off
  Average age : Outport  Port=2  VectorParamsAs1DForOutWhenUnconnected=off
  wires:
  Sum/1 -> Growth: max growth is max volume minus current volume minus losses./1
  Max volume/1 -> Sum/1
  Growth: max growth is max volume minus current volume minus losses./1 -> "Growth "/1
  AGE/1(Average age) -> Average age/1, Average growth m3/ha/1
  Volume/1 -> Sum/3, AGE/1(Volume)
  Product/1 -> Growth: max growth is max volume minus current volume minus losses./2
  Average growth m3/ha/1 -> Product/1
  Area (ha)/1 -> Product/2
  "Final felling and natural loss "/1 -> Sum1/1, AGE/2(Final felling and natural loss)
  Thinning/1 -> Sum1/2
  Sum1/1 -> Sum/2
  Constant/1 -> Growth: max growth is max volume minus current volume minus losses./3

== system carboncycle/FOREST/Initial stock ==
  In1 : Inport
  Action Port : ActionPort  ActionPortLabel=if(u1 < 0)
  Out1 : Outport
  wires:
  In1/1 -> Out1/1

== system carboncycle/FOREST/Initial stock1 ==
  In1 : Inport
  Action Port : ActionPort  ActionPortLabel=if(u1 < 0)
  Out1 : Outport
  wires:
  In1/1 -> Out1/1

== system carboncycle/FOREST/GROWING/AGE ==
  note: The average age increases
      | by one year for those not
      | harvested.
  note: If final fell + natural loss is x% (from current volume), the average age decreases by x% (not sure if realistic, though).
  Volume : Inport
  Final felling and natural loss : Inport  Port=2
  Age : Integrator  InitialCondition=forest_age_0
  Constant : Constant
  Divide : Product  Inputs=*/
  Product : Product
  Sum : Sum  Inputs=-+|
  Average age : Outport  VectorParamsAs1DForOutWhenUnconnected=off
  wires:
  Divide/1 -> Product/1
  Product/1 -> Sum/1
  Constant/1 -> Sum/2
  Sum/1 -> Age/1
  Final felling and natural loss/1 -> Divide/1
  Volume/1 -> Divide/2
  Age/1 -> Average age/1, Product/2
